simulink model "MITLungWorking_NC"  (R2020a)
settings: Solver=ode23tb  StartTime=0.0  StopTime=30  MaxStep=0.1  MinStep=1e-16  RelTol=1e-8  AbsTol=1e-9
PostLoadFcn:
  | hws = get_param(bdroot, 'modelworkspace');
  | hws.assignin('T_room', 20); % degC
  | hws.assignin('RH_room', 0.1); % degC
  | hws.assignin('T_humidifier', 40); % degC
  | hws.assignin('T_body', 37); % degC
  | 
  | hws.assignin('L_tube', 1); % m
  | hws.assignin('D_tube', 0.01); % m
  | hws.assignin('L_trachea', 0.15); % m
  | hws.assignin('D_trachea', 0.015); % m
  | 
  | % Conversion factors
  | hws.assignin('cmH2O_to_Pa', 98.0665);
  | hws.assignin('L_to_m3', 1e-3);
  | 
  | % L Functional Residual Capacity https://www.ncbi.nlm.nih.gov/books/NBK500007/
  | hws.assignin('FRC', 2);
  | hws.assignin('P_muscle', 0); % cmH2O
  | %E_respiratory = 20; % cmH2O/L    C_respiratory = 1/E_respiratory * 1000;
  | % http://www.ubccriticalcaremedicine.ca/rotating/material/Lecture_1%20for%20Residents.pdf
  | 
  | clear hws;
StopFcn:
  | fileExisting = (exist('Lung_Simulation_Data.xls', 'file') == 2);
  | col_header = {'TAIP (ms)','Respiratory Rate (breaths/min)','I:E Ratio','Target Peak Pressure (cm H2O)','Observed Peak Pressure (cm H2O)','PEEP (cm H2O)', 'Lung Compliance (mL / cm H2O)', 'Airway Resistance (cm H2O / (L/s) )','Tidal Volume (mL)', 'Flow (L/min)'};
  | index = 0;
  | if fileExisting == 0
  | xlswrite('Lung_Simulation_Data.xls',col_header,'Sheet1','A1:J1');
  | index = 2;
  | else
  | read_xls = xlsread('Lung_Simulation_Data.xls');
  | [file_rows file_cols] = size(read_xls);
  | index = file_rows + 2;
  | end
  | if index == 0
  | xlswrite('Lung_Simulation_Data.xls', col_header,0,0);
  | index = 2;
  | end
  | tidal_volume_data = max(tidal_volume_info.signals(1).values) - min(tidal_volume_info.signals(1).values);
  | observed_pressure_data = max(observed_pressure_info.signals(1).values) - min(observed_pressure_info.signals(1).values);
  | Flow_data_max = max(FlowData.signals(1).values);
  | table_data = [getdatasamples(TAIPdata, [1]), getdatasamples(RRdata,[1]), getdatasamples(IEdata,[1]) , getdatasamples(IPdata, [1]), observed_pressure_data(1), getdatasamples(PEEPdata, [1]), getdatasamples(Compdata, [1]), getdatasamples(Resdata, [1]), tidal_volume_data, Flow_data_max];
  | col_start = 'A';
  | col_end = 'J';
  | row_start = index;
  | row_end = row_start;
  | input_data_range = [col_start,num2str(row_start),':',col_end,num2str(row_end)];
  | writematrix(table_data, 'Lung_Simulation_Data.xls', 'Sheet', 1, 'Range', input_data_range);
  | 
  | LungVData = LungVData.signals(1).values;
  | TVData = TVdata.signals(1).values;
  | FlowData = FlowData.signals(1).values;
  | PressureData = PressureData.signals(1).values;
  | 
  | LungVDataFile = ['Lung_Simulation_LungVData',num2str(total_runs)];
  | TVDataFile = ['Lung_Simulation_TVData',num2str(total_runs)];
  | FlowDataFile = ['Lung_Simulation_FlowData',num2str(total_runs)];
  | PressureDataFile = ['Lung_Simulation_PressureData',num2str(total_runs)];
  | 
  | writematrix(LungVData, LungVDataFile);
  | writematrix(TVData, TVDataFile);
  | writematrix(FlowData, FlowDataFile);
  | writematrix(PressureData, PressureDataFile);
model workspace (MAT data in the model file):
  C_respiratory = 10
  D_trachea = 0.015
  D_tube = 0.01
  FRC = 2
  IE = 2
  L_to_m3 = 0.001
  L_trachea = 0.15
  L_tube = 1
  P_muscle = 0
  RH_room = 0.1
  R_respiratory = 1
  RunNum = 2
  Sig : Simulink.Signal (value not decoded)
  TAIP = 2000
  T_body = 37
  T_humidifier = 40
  T_period = 5
  T_room = 20
  cmH2O_to_Pa = 98.0665
  input_pressure = 20
  minute_volume = 0
  p_crack = 5
  pressure_increment = 0
  respiratory_rate = 12
values from neighbouring files (symbols this model uses):
  total_runs = total_runs - 1    [RunLungSimulation.m]
libraries: fl_lib x42, nesl_utility x8, simulink x3
(part 2 of 2)

== matlab function MITLungWorking_NC/Pressure Source/Pressure Waveform Generator ==
  data: t input; Vent_Pressure output; Valve_Flow output; respiratory_rate parameter; IE parameter; input_pressure parameter; D_tube parameter; TAIP parameter; TAIPdata output; RRdata output; IPdata output; IEdata output; T_period parameter
function [Vent_Pressure, Valve_Flow, TAIPdata, RRdata, IPdata, IEdata] = fcn(t, respiratory_rate, IE, input_pressure, D_tube, TAIP, T_period)

%Time constants
TAIP = TAIP/1000;
input_pressure = (input_pressure)*98.0665;
T_inspiration = 1/(IE+1) * T_period;
T_inhale_hold = 0.1; 
cycle_timer = rem(t,T_period);
inhale = 0;
exhale = 0;
duration = (T_inspiration - T_inhale_hold);
if TAIP == 0
    if cycle_timer <= duration
        inhale = 1;
        exhale = 0;
    elseif cycle_timer > T_inspiration
        inhale = 0;
        exhale = 1;
    else
        inhale = 0;
        exhale = 0;
    end
elseif TAIP > 0
    if cycle_timer <= duration
        if cycle_timer <= TAIP
            slope = 1/TAIP;
            t = cycle_timer - 0;
            inhale = slope*t;
        else
            slope = 1;
            t = cycle_timer - T_inspiration;
            inhale = slope;
        end
        exhale = 0;
    elseif cycle_timer > T_inspiration
        inhale = 0;
        exhale = 1;
    end
end
MaxValveArea = pi*D_tube^2/4;
TAIPdata = TAIP*1000;
RRdata = respiratory_rate;
IPdata = input_pressure/98.0665;
IEdata = IE;
Vent_Pressure = inhale*input_pressure;
Valve_Flow = MaxValveArea * exhale;
